simulink library "xrbsControl_r4"  (Simulink 7.1)
undefined symbols (not defined in the file or in its folder): xlDistRamDepth, xlMatrixToOutputVec, xlMatrixToStateInitVec, xlNumMealyElements, xlNumMooreOutputElements, xlNumMooreStateElements, xlNumStateBits, xlRegMealyInitVec
libraries: xbsIndex_r4 x13
settings Model: Creator=singhj  LastModifiedBy=sysgengroup

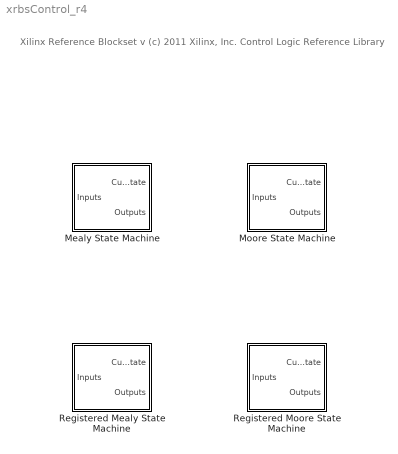
== system xrbsControl_r4 ==
  note: Xilinx Reference Blockset v
      | (c) 2011 Xilinx, Inc.
      |
      | Control Logic Reference Library
  Mealy State Machine : Subsystem  mask(Xilinx Mealy State Machine){next_state_matrix=[0 1; 2 1; 0 3; 2 1], output_matrix=[0 0; 0 0; 0 0; 0 1], n_bits=1, period=1}
      mask prompts: next_state_matrix "Next State Matrix"; output_matrix "Output Matrix"; n_bits "Number of  Output Bits"; period "Sample Period"
      mask help: Implements a Mealy state machine. The output is a function of the current state and input.
      mask init:
      | % Set Block Logo
      | [bg,fg] = xlcmap('XBlock',0);
      | iPos = get_param(gcb,'Position');
      | iWidth=iPos(3)-iPos(1); iHeight=iPos(4)-iPos(2);
      | iCx=iWidth/2;
      | iCy=iHeight/2;
      | [logoX, logoY] = xlogo(iPos);
      mask Help: eval('');xlDoc('-book','sysgen','-topic','Mealy_State_Machine');
      mask Display:
      | patch([0 iWidth iWidth 0],[0 0 iHeight iHeight] , bg);
      | patch(logoX,logoY, fg);
      | port_label('input',1,'Inputs');
      | port_label('output',1,'CurrentState');
      | port_label('output',2,'Outputs');
      | 
      | plot([0 0 iWidth iWidth 0], [0 iHeight iHeight 0 0]);
  Moore State Machine : Subsystem  mask(Xilinx Moore State Machine){next_state_matrix=[0 1; 2 1; 0 3; 2 4; 0 1], output_matrix=[0; 0; 0; 0; 1], n_bits=1, period=1}
      mask prompts: next_state_matrix "Next State Matrix"; output_matrix "Output Array"; n_bits "Number of Output Bits"; period "Sample Period"
      mask help: Implements a Moore state machine. The output is a function only of the current state.
      mask init:
      | % Set Block Logo
      | [bg,fg] = xlcmap('XBlock',0);
      | iPos = get_param(gcb,'Position');
      | iWidth=iPos(3)-iPos(1); iHeight=iPos(4)-iPos(2);
      | iCx=iWidth/2;
      | iCy=iHeight/2;
      | [logoX, logoY] = xlogo(iPos);
      mask Help: eval('');xlDoc('-book','sysgen','-topic','Moore_State_Machine');
      mask Display:
      | patch([0 iWidth iWidth 0],[0 0 iHeight iHeight] , bg);
      | patch(logoX,logoY, fg);
      | port_label('input',1,'Inputs');
      | port_label('output',1,'CurrentState');
      | port_label('output',2,'Outputs');
      | 
      | plot([0 0 iWidth iWidth 0], [0 iHeight iHeight 0 0]);
  Registered Mealy State Machine : Subsystem  mask(Xilinx Registered Mealy State Machine){next_state_matrix=[0 1; 2 1; 0 3; 2 1], output_matrix=[0 0; 0 0; 0 0; 0 1], n_bits=1, period=1}
      mask prompts: next_state_matrix "Next State Matrix"; output_matrix "Output Matrix"; n_bits "Number of Output Bits"; period "Sample Period"
      mask help: Implements a registered Mealy state machine. The output is a function of the current state and its input. The output is registered.
      mask init:
      | % Set Block Logo
      | [bg,fg] = xlcmap('XBlock',0);
      | iPos = get_param(gcb,'Position');
      | iWidth=iPos(3)-iPos(1); iHeight=iPos(4)-iPos(2);
      | iCx=iWidth/2;
      | iCy=iHeight/2;
      | [logoX, logoY] = xlogo(iPos);
      mask Help: eval('');xlDoc('-book','sysgen','-topic','Registered_Mealy_State_Machine');
      mask Display:
      | patch([0 iWidth iWidth 0],[0 0 iHeight iHeight] , bg);
      | patch(logoX,logoY, fg);
      | port_label('input',1,'Inputs');
      | port_label('output',1,'CurrentState');
      | port_label('output',2,'Outputs');
      | 
      | plot([0 0 iWidth iWidth 0], [0 iHeight iHeight 0 0]);
  Registered Moore State Machine : Subsystem  mask(Xilinx Registered Moore State Machine){next_state_matrix=[0 1; 2 1; 0 3; 2 4; 0 1], output_matrix=[0; 0; 0; 0; 1], n_bits=1, period=1}
      mask prompts: next_state_matrix "Next State Matrix"; output_matrix "Output Array"; n_bits "Number of Output Bits"; period "Sample Period"
      mask help: Implements a registered Moore state machine. The output is a function only of the current state. The output is registered.
      mask init:
      | % Set Block Logo
      | [bg,fg] = xlcmap('XBlock',0);
      | iPos = get_param(gcb,'Position');
      | iWidth=iPos(3)-iPos(1); iHeight=iPos(4)-iPos(2);
      | iCx=iWidth/2;
      | iCy=iHeight/2;
      | [logoX, logoY] = xlogo(iPos);
      mask Help: eval('');xlDoc('-book','sysgen','-topic','Registered_Moore_State_Machine');
      mask Display:
      | patch([0 iWidth iWidth 0],[0 0 iHeight iHeight] , bg);
      | patch(logoX,logoY, fg);
      | port_label('input',1,'Inputs');
      | port_label('output',1,'CurrentState');
      | port_label('output',2,'Outputs');
      | 
      | plot([0 0 iWidth iWidth 0], [0 iHeight iHeight 0 0]);

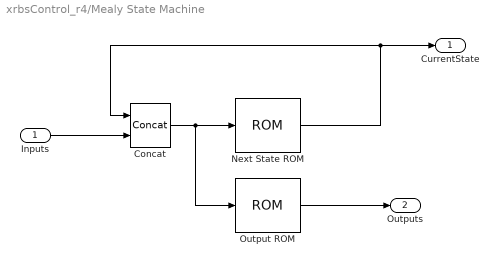
== system xrbsControl_r4/Mealy State Machine ==
  Inputs : Inport  OutDataType=sfix(16)  OutScaling=2^0
  Concat : xbsIndex_r4/Concat  num_inputs=2  dbl_ovrd=off  block_type=concat
      settings: block_version=VER_STRING_GOES_HERE
  Next State ROM : xbsIndex_r4/ROM  depth=xlNumMealyElements(next_state_matrix, output_matrix)  initVector=xlMatrixToStateInitVec(next_state_matrix,xlNumStateBits(next_state_matrix),0,1,1,1)  rst=off  init_reg=0  en=off  latency=1  arith_type=Unsigned  n_bits=xlNumStateBits(next_state_matrix)  bin_pt=0  dbl_ovrd=off  distributed_mem=Block RAM  use_rpm=off  block_type=sprom
      settings: xl_area=[0, 0, 0, 0, 0, 0, 0]  block_version=VER_STRING_GOES_HERE
  Output ROM : xbsIndex_r4/ROM  depth=xlDistRamDepth(output_matrix)  initVector=xlMatrixToOutputVec(output_matrix,n_bits,0,1,1,1)  rst=off  init_reg=0  en=off  latency=0  arith_type=Unsigned  n_bits=n_bits  bin_pt=0  dbl_ovrd=off  distributed_mem=Distributed memory  use_rpm=off  block_type=sprom
      settings: xl_area=[0, 0, 0, 0, 0, 0, 0]  block_version=VER_STRING_GOES_HERE
  CurrentState : Outport  OutDataType=sfix(16)  OutScaling=2^0
  Outputs : Outport  Port=2  OutDataType=sfix(16)  OutScaling=2^0
  wires:
  Inputs/1 -> Concat/2
  Output ROM/1 -> Outputs/1
  Concat/1 -> Next State ROM/1, Output ROM/1
  Next State ROM/1 -> Concat/1, CurrentState/1

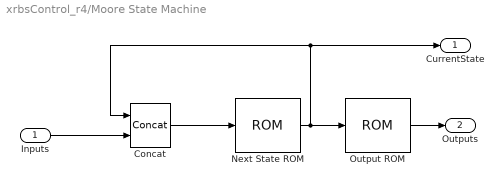
== system xrbsControl_r4/Moore State Machine ==
  Inputs : Inport  OutDataType=sfix(16)  OutScaling=2^0
  Concat : xbsIndex_r4/Concat  num_inputs=2  dbl_ovrd=off  block_type=concat
      settings: block_version=VER_STRING_GOES_HERE
  Next State ROM : xbsIndex_r4/ROM  depth=xlNumMooreStateElements(next_state_matrix, output_matrix)  initVector=xlMatrixToStateInitVec(next_state_matrix,xlNumStateBits(next_state_matrix),0,1,1,1)  rst=off  init_reg=0  en=off  latency=1  arith_type=Unsigned  n_bits=xlNumStateBits(next_state_matrix)  bin_pt=0  dbl_ovrd=off  distributed_mem=Block RAM  use_rpm=off  block_type=sprom
      settings: xl_area=[0, 0, 0, 0, 0, 0, 0]  block_version=VER_STRING_GOES_HERE
  Output ROM : xbsIndex_r4/ROM  depth=xlDistRamDepth(output_matrix)  initVector=xlMatrixToOutputVec(output_matrix,n_bits,0,1,1,1)  rst=off  init_reg=0  en=off  latency=0  arith_type=Unsigned  n_bits=n_bits  bin_pt=0  dbl_ovrd=off  distributed_mem=Distributed memory  use_rpm=off  block_type=sprom
      settings: xl_area=[0, 0, 0, 0, 0, 0, 0]  block_version=VER_STRING_GOES_HERE
  CurrentState : Outport  OutDataType=sfix(16)  OutScaling=2^0
  Outputs : Outport  Port=2  OutDataType=sfix(16)  OutScaling=2^0
  wires:
  Inputs/1 -> Concat/2
  Output ROM/1 -> Outputs/1
  Concat/1 -> Next State ROM/1
  Next State ROM/1 -> Concat/1, CurrentState/1, Output ROM/1

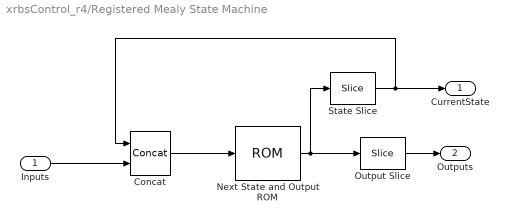
== system xrbsControl_r4/Registered Mealy State Machine ==
  Inputs : Inport  OutDataType=sfix(16)  OutScaling=2^0
  Concat : xbsIndex_r4/Concat  num_inputs=2  dbl_ovrd=off  block_type=concat
      settings: block_version=VER_STRING_GOES_HERE
  Next State and Output ROM : xbsIndex_r4/ROM  depth=xlNumMealyElements(next_state_matrix, output_matrix)  initVector=xlRegMealyInitVec(next_state_matrix, output_matrix, n_bits,0,1,1,1)  rst=off  init_reg=0  en=off  latency=1  arith_type=Unsigned  n_bits=xlNumStateBits(next_state_matrix)+n_bits  bin_pt=0  dbl_ovrd=off  distributed_mem=Block RAM  use_rpm=off  block_type=sprom
      settings: xl_area=[0, 0, 0, 0, 0, 0, 0]  block_version=VER_STRING_GOES_HERE
  Output Slice : xbsIndex_r4/Slice  nbits=n_bits  boolean_output=off  mode=Lower Bit Location + Width  bit1=0  base1=MSB of Input  bit0=0  base0=LSB of Input  dbl_ovrd=off  block_type=slice
      settings: infoedit="Extracts a given range of bits from each input sample and presents it at the output.  The output type is ordinarily unsigned with binary point at zero, but can be Boolean when the slice is one bit wide.<P><P>Hardware notes: In hardware this block costs nothing."  block_version=VER_STRING_GOES_HERE
  State Slice : xbsIndex_r4/Slice  nbits=xlNumStateBits(next_state_matrix)  boolean_output=off  mode=Upper Bit Location + Width  bit1=0  base1=MSB of Input  bit0=0  base0=LSB of Input  dbl_ovrd=off  block_type=slice
      settings: infoedit="Extracts a given range of bits from each input sample and presents it at the output.  The output type is ordinarily unsigned with binary point at zero, but can be Boolean when the slice is one bit wide.<P><P>Hardware notes: In hardware this block costs nothing."  block_version=VER_STRING_GOES_HERE
  CurrentState : Outport  OutDataType=sfix(16)  OutScaling=2^0
  Outputs : Outport  Port=2  OutDataType=sfix(16)  OutScaling=2^0
  wires:
  Inputs/1 -> Concat/2
  Output Slice/1 -> Outputs/1
  Concat/1 -> Next State and Output ROM/1
  Next State and Output ROM/1 -> Output Slice/1, State Slice/1
  State Slice/1 -> CurrentState/1, Concat/1

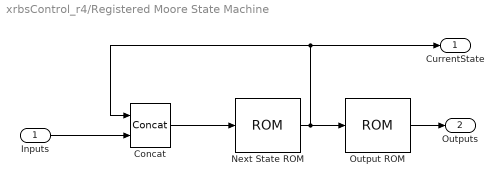
== system xrbsControl_r4/Registered Moore State Machine ==
  Inputs : Inport  OutDataType=sfix(16)  OutScaling=2^0
  Concat : xbsIndex_r4/Concat  num_inputs=2  dbl_ovrd=off  block_type=concat
      settings: block_version=VER_STRING_GOES_HERE
  Next State ROM : xbsIndex_r4/ROM  depth=xlNumMooreStateElements(next_state_matrix, output_matrix)  initVector=xlMatrixToStateInitVec(next_state_matrix,xlNumStateBits(next_state_matrix),0,1,1,1)  rst=off  init_reg=0  en=off  latency=1  arith_type=Unsigned  n_bits=xlNumStateBits(next_state_matrix)  bin_pt=0  dbl_ovrd=off  distributed_mem=Block RAM  use_rpm=off  block_type=sprom
      settings: xl_area=[0, 0, 0, 0, 0, 0, 0]  block_version=VER_STRING_GOES_HERE
  Output ROM : xbsIndex_r4/ROM  depth=xlNumMooreOutputElements(output_matrix)  initVector=xlMatrixToOutputVec(output_matrix,n_bits,0,1,1,1)  rst=off  init_reg=0  en=off  latency=1  arith_type=Unsigned  n_bits=n_bits  bin_pt=0  dbl_ovrd=off  distributed_mem=Block RAM  use_rpm=off  block_type=sprom
      settings: xl_area=[0, 0, 0, 0, 0, 0, 0]  block_version=VER_STRING_GOES_HERE
  CurrentState : Outport  OutDataType=sfix(16)  OutScaling=2^0
  Outputs : Outport  Port=2  OutDataType=sfix(16)  OutScaling=2^0
  wires:
  Next State ROM/1 -> Output ROM/1, CurrentState/1, Concat/1
  Concat/1 -> Next State ROM/1
  Output ROM/1 -> Outputs/1
  Inputs/1 -> Concat/2
